simulink model "Correccion_Sist_Fisico"  (R2021a)
settings: Solver=VariableStepAuto  StartTime=0.0  StopTime=inf  RelTol=1e-3
values from neighbouring files (symbols this model uses):
  b_cx = 1*10^6    (= 1000000)    [parametros.m]
  b_cy = 1*10^7    (= 10000000)    [parametros.m]
  b_eq = (b_td+b_tm*(r_t^2))/r_td    (= 10803.6)    [parametros.m]
  b_eqh = 2*(b_hd+b_hm*(r_h^2))/r_hd    (= 23253.3333333)    [parametros.m]
  b_ha = b_eqh/r_h - n_h*w_posh*(J_eqh + 0.5*m_l_*r_hd)/r_h    [parametros.m]
  b_hb = 1*10^8    (= 100000000)    [parametros.m]
  b_hEb = 2.2*10^9    (= 2200000000)    [parametros.m]
  b_t = 90    [parametros.m]
  b_ta = n_t*w_post*(r_td*J_eqt/r_t) - r_td*b_eqt/r_t    [parametros.m]
  b_tb = 5*10^6    (= 5000000)    [parametros.m]
  b_tw = 3*10^3    (= 3000)    [parametros.m]
  b_wu = 150    [parametros.m]
  g = 9.80665    [parametros.m]
  H_c = 2.5    [parametros.m]
  J_eq = (J_td+J_tm_tb*(r_t^2))/r_td    (= 15000)    [parametros.m]
  J_eqh = 2*(J_hd_hEb+J_hm_hb*(r_h^2))/r_hd    (= 48853.3333333)    [parametros.m]
  K_cy = 1.8*10^9    (= 1800000000)    [parametros.m]
  K_hsa = -n_h*(w_posh^2)*(J_eqh + 0.5*m_l_*r_hd)/r_t    [parametros.m]
  K_hsia = -(w_posh^3)*(J_eqh + 0.5*m_l_*r_hd)/r_t    [parametros.m]
  K_tsa = n_t*(w_post^2)*J_eqt*r_td/r_t    [parametros.m]
  K_tsia = (w_post^3)*J_eqt*r_td/r_t    [parametros.m]
  K_tw = 4.8*10^5    (= 480000)    [parametros.m]
  k_wu = 2.36*10^8    (= 236000000)    [parametros.m]
  lh_inicial = 45-yl_inicial    (= 40)    [parametros.m]
  M_c_MAX = 50000 + M_s    (= 65000)    [parametros.m]
  M_real = 10000    [parametros.m]
  M_s = 15000    [parametros.m]
  M_t = 30000    [parametros.m]
  r_h = 22    [parametros.m]
  r_hd = 0.75    [parametros.m]
  r_t = 30    [parametros.m]
  r_td = 0.5    [parametros.m]
  T_hb_MAX = 5*10^4    (= 50000)    [parametros.m]
  T_hEb_MAX = 1.1*10^6    (= 1100000)    [parametros.m]
  T_hm_MAX = 2*10^4    (= 20000)    [parametros.m]
  T_s2 = 5e-3    (= 0.005)    [parametros.m]
  T_tb_MAX = 5*10^3    (= 5000)    [parametros.m]
  T_tm_MAX = 3*10^3    (= 3000)    [parametros.m]
  tau_hm = 1.0e-2    (= 0.01)    [parametros.m]
  tau_tm = 1.0e-2    (= 0.01)    [parametros.m]
  TensionMinima = (M_s*g/2)*0.5    (= 36774.9375)    [parametros.m]
  v_h_MAX_c = +1.5    (= 1.5)    [parametros.m]
  v_t_MAX = +4    (= 4)    [parametros.m]
  v_t_MIN = -4    [parametros.m]
  w_hm_min = pi/4    (= 0.785398163397)    [parametros.m]
  w_tm_min = pi/4    (= 0.785398163397)    [parametros.m]
  xt_inicial = -10    [parametros.m]
  Y_t0 = 45    [parametros.m]
  yl_inicial = 5    [parametros.m]
undefined symbols (not defined in the file or in its folder): DiscIntNeverNeededParam
libraries: simulink x10, dspstat3 x1, vrlib x1
(part 2 of 3)

== matlab function Correccion_Sist_Fisico/Estimacion de Masa/MATLAB Function1 ==
  settings: updateMethod=DISCRETE
  data: tension input; dF_hw input; m_l output; M_cX output; TLK input; MasaFija output
function [m_l, M_cX, MasaFija] = fcn(tension,dF_hw, TLK)

%--------------------------------------------------------------------------%
%---------------------Declaracion variables PERSISTENT---------------------% 
%--------------------------------------------------------------------------%
            % --> Persistent: local variable in a function that retains its 
                            % value in memory between calls to the function
    persistent masaPromedio
    persistent contador
    persistent masaEnclavada
    persistent masaFijada
    
    persistent Masa_Spreader
    persistent Peso_Spreader

%--------------------------------------------------------------------------%
%------------------Inicialización de variables PERSISTENT------------------% 
%--------------------------------------------------------------------------%
    if isempty(masaPromedio)
        masaPromedio = zeros(1, 5);
    end
    if isempty(contador)
        contador = 0;
    end
    if isempty(masaEnclavada)
        masaEnclavada = 0;
    end
    if isempty(masaFijada)
        masaFijada = 0;
    end
    if isempty(Masa_Spreader)
        Masa_Spreader = 15000; % Kg
    end
    if isempty(Peso_Spreader)
        Peso_Spreader = Masa_Spreader * 9.8;
    end
    
%--------------------------------------------------------------------------%
%-----------------------------Lógica principal-----------------------------%
%--------------------------------------------------------------------------%

    if TLK == 1 && masaEnclavada == 0             % Si la masa ya está enclavada no vuelve a entrar para evitar que variaciones en la tensión afecten
        if dF_hw<10 && tension >= Peso_Spreader*1.1            % Peso Spreader + 10%
            m_l = tension * 2 / 9.81;             % El 2 es por la polea
            M_cX = m_l - Masa_Spreader;
            MasaFija = 0;                         % Valor booleano de salida 
            contador = contador + 1;
 
            if contador > length(masaPromedio)    % Por lo menos 100 masas para calcular el promedio
                masaPromedio(1:4) = masaPromedio(2:end);
                masaPromedio(end) = m_l;
                promedio = sum(masaPromedio) / length(masaPromedio);

                if promedio < (m_l + 1000) && promedio > (m_l - 1000)
                    masaEnclavada = 1;
                    masaFijada = m_l;
                    MasaFija = 1;
                end
            else
                masaPromedio(contador) = m_l;
            end
        else
            m_l = 35000;                    % Valor inicial de masa (Promedio entre Max y Min + Spreader)
            M_cX = m_l - Masa_Spreader;
            MasaFija = 0;
        end
    elseif TLK == 0
        masaEnclavada = 0;
        contador = 0;
        m_l = Masa_Spreader ;
        M_cX = m_l - Masa_Spreader;
        MasaFija = 1;
    elseif masaEnclavada == 1
        m_l = masaFijada;
        M_cX = m_l - Masa_Spreader;
        MasaFija = 1;
    else 
        m_l=Masa_Spreader;
        M_cX = 0;
        MasaFija=0;
    end
end

== stateflow chart Correccion_Sist_Fisico/Nivel 0: Seguridad o Proteccion ==
  state Nivel_0_Encendido
    state Espera
      entry:
      Emergencia = 0;
      BRK_t = 1;
      BRK_h = 1;
      BRK_hE = 1;
      Ciclos = 0;
      state FINES_DE_CARRERA_ULTIMOS [parallel]
        settings: executionOrder=2
        state Fin_AV_Carro
          entry:
          Emergencia = 2;
        state Espera
        state Fin_AV_Izaje
          entry:
          Emergencia = 3;
        (default) -> Nivel_0_Encendido.Espera.FINES_DE_CARRERA_ULTIMOS.Espera
        Nivel_0_Encendido.Espera.FINES_DE_CARRERA_ULTIMOS.Espera -> Fin_AV_Carro [order 1] : [Fin_Der_u || Fin_Izq_u ]
        Nivel_0_Encendido.Espera.FINES_DE_CARRERA_ULTIMOS.Espera -> Fin_AV_Izaje [order 2] : [Fin_Sup_u || Fin_Inf_u ]
      state BOTON_EMERGENCIA [parallel]
        settings: executionOrder=1
        state Espera
        state Emergencia
          entry:
          Emergencia = 1;
        (default) -> Nivel_0_Encendido.Espera.BOTON_EMERGENCIA.Espera
        Nivel_0_Encendido.Espera.BOTON_EMERGENCIA.Espera -> Emergencia : [Boton_Emergencia == 1]
      state VIDA_WATCHDOG [parallel]
        settings: executionOrder=3
        state Espera
        state Contador_Ciclos
          entry:
          Ciclos = Ciclos + 1;
        state Hay_Vida
          entry:
          Ciclos = 0;
        state No_Vida
          entry:
          Emergencia = 1;
        (default) -> Nivel_0_Encendido.Espera.VIDA_WATCHDOG.Espera
        Nivel_0_Encendido.Espera.VIDA_WATCHDOG.Espera -> Contador_Ciclos [order 1] : after(550,msec)
        Contador_Ciclos -> Nivel_0_Encendido.Espera.VIDA_WATCHDOG.Espera [order 2]
        Hay_Vida -> Nivel_0_Encendido.Espera.VIDA_WATCHDOG.Espera
        Nivel_0_Encendido.Espera.VIDA_WATCHDOG.Espera -> Hay_Vida [order 2] : [Vida == 1]
        Contador_Ciclos -> No_Vida [order 1] : [Ciclos == 3]
      state SOBREVELOCIDAD [parallel]
        settings: executionOrder=4
        state Espera
        state Sobrevelocidad_Izaje
          entry:
          Emergencia = 0;
        (default) -> Nivel_0_Encendido.Espera.SOBREVELOCIDAD.Espera
        Nivel_0_Encendido.Espera.SOBREVELOCIDAD.Espera -> Sobrevelocidad_Izaje : [abs(w_hm)>=1.5*abs(w_hm_max)]
    note: --> El nivel 1 deberia mandar señales de vida
        |      cada 500 msec. Si por más de 3 ciclos no manda señales entra en
        |      modo de emergencia
    state Mover_IZAJE1
      entry:
      BRK_t = 1;
    state Emergencia_CARRO
      entry:
      BRK_t = 0;
    state Emergencia_TOTAL
      entry:
      BRK_t = 0;
      BRK_h = 0;
      BRK_hE = 0;
    state Emergencia_IZAJE
      entry:
      BRK_h = 0;
      BRK_hE = 0;
    state Mover_IZAJE
      entry:
      BRK_h = 1;
      BRK_hE = 1;
    note: CAMBIE ESTO A 0 PORQUE ME DABA UN ERROR YA QUE SE VUELVE LOCO PORQUE HAY QUE PONERLE LAS CONDICIONES ACA AL LADO
    (default) -> Nivel_0_Encendido.Espera
    Nivel_0_Encendido.Espera -> Emergencia_CARRO [order 2] : [Emergencia == 2]
    Emergencia_CARRO -> Mover_IZAJE1 [order 2] : [(dx_t_ref_man < 0 && Fin_Der_u) || (dx_t_ref_man > 0 && Fin_Izq_u)]
    Mover_IZAJE1 -> Emergencia_CARRO : [(dx_t_ref_man >= 0 && Fin_Der_u) || (dx_t_ref_man <= 0 && Fin_Inf_u) || (~Fin_Der_u && ~Fin_Izq_u)]
    Emergencia_CARRO -> Nivel_0_Encendido.Espera [order 1] : [Fin_Der_u == 0 &&  Fin_Izq_u  == 0  ]
    Emergencia_TOTAL -> Nivel_0_Encendido.Espera : [Boton_Emergencia == 0 && Vida == 1]
    Nivel_0_Encendido.Espera -> Emergencia_TOTAL [order 1] : [Emergencia == 1]
    Nivel_0_Encendido.Espera -> Emergencia_IZAJE [order 3] : [Emergencia == 3]
    Emergencia_IZAJE -> Mover_IZAJE [order 2] : [(dl_h_ref_man > 0 && Fin_Sup_u) || (dl_h_ref_man < 0 && Fin_Inf_u)]
    Mover_IZAJE -> Emergencia_IZAJE : [(dl_h_ref_man <= 0 && Fin_Sup_u) || (dl_h_ref_man >= 0 && Fin_Inf_u) || (~Fin_Sup_u && ~Fin_Inf_u)]
    Emergencia_IZAJE -> Nivel_0_Encendido.Espera [order 1] : [Fin_Sup_u == 0 && Fin_Inf_u == 0]
  state Nivel_0_Apagado
  (default) -> Nivel_0_Apagado
  Nivel_0_Apagado -> Nivel_0_Encendido : [Encendido_Nivel_0 == 1]
  Nivel_0_Encendido -> Nivel_0_Apagado : [Encendido_Nivel_0 == 0]
  data: Boton_Emergencia input; BRK_t output; BRK_h output; BRK_hE output; Fin_Der_u input; Fin_Izq_u input; Fin_Sup_u input; Fin_Inf_u input; Vida input; Emergencia output size=1; Encendido_Nivel_0 input; w_hm input; Ciclos local; w_hm_max parameter; dl_h_ref_man input; dx_t_ref_man input
